simulink model "mpc1_sim_extended"  (R2020a)
settings: Solver=VariableStepAuto  StartTime=0.0  StopTime=10  RelTol=1e-3
values from neighbouring files (symbols this model uses):
  Ts = 0.1    [data_mpc.mat]    (also in so_priklad.m)
libraries: mpclib x3, cstblocks x3
settings Model: Creator=mgoubej  LastModifiedBy=mgoubej

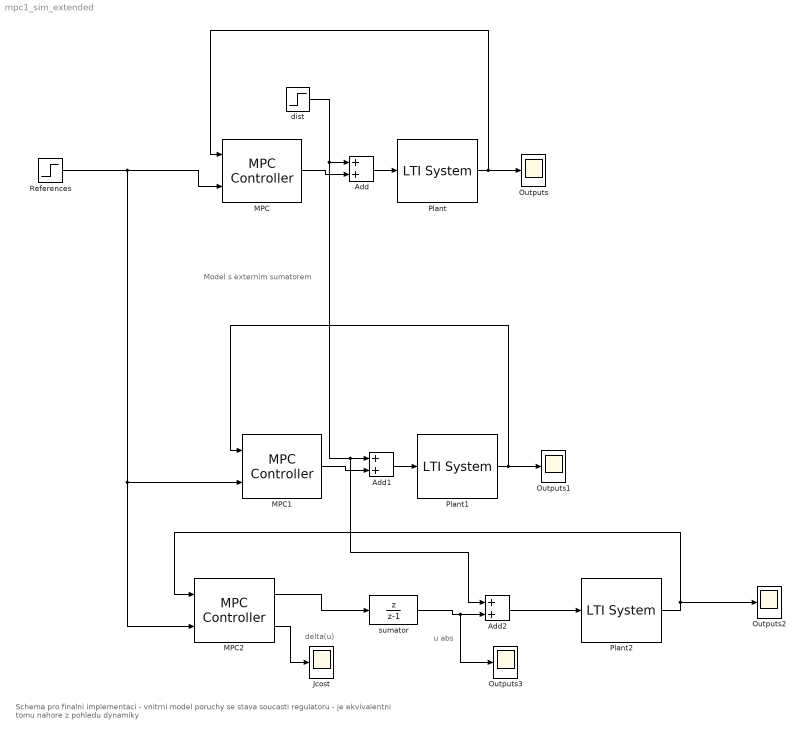
== system mpc1_sim_extended ==
  note: Schema pro finalni implementaci - vnitrni model poruchy se stava soucasti regulatoru - je ekvivalentni tomu nahore z pohledu dynamiky
  note: u abs
  note: delta(u)
  note: Model s externim sumatorem
  Add : Sum
  Add1 : Sum
  Add2 : Sum
  Jcost : Scope
  MPC : mpclib/MPC Controller  SCDEnableBlockLinearizationSpecification=on  mpcobj=mpc1_e  is_multiple=0  enable_value=0  return_u0=off  updateMPCinCallerWorkspace=on  md_inport=off  mv_inport=off  uref_inport=off  return_cost=off  return_mvseq=off  return_qpstatus=off  return_xseq=off  return_state=off  return_ovseq=off  state_inport=off  umin_inport=off  umax_inport=off  ymin_inport=off  ymax_inport=off  cc_inport=off  ywt_inport=off  uwt_inport=off  duwt_inport=off  rhoeps_inport=off  pm_inport=off  MaximumP=10  HorizonChoice=FixedHorizon  n_ts=0.1  n_p=10  n_mv=1  n_md=0  n_ud=0  n_mo=1  n_uo=0  BlockDataType=double  SampleTimeInherited=off  switch_inport=off
  MPC1 : mpclib/MPC Controller  SCDEnableBlockLinearizationSpecification=on  mpcobj=mpc1_e  is_multiple=0  enable_value=0  return_u0=off  updateMPCinCallerWorkspace=on  md_inport=off  mv_inport=off  uref_inport=off  return_cost=off  return_mvseq=off  return_qpstatus=off  return_xseq=off  return_state=off  return_ovseq=off  state_inport=off  umin_inport=off  umax_inport=off  ymin_inport=off  ymax_inport=off  cc_inport=off  ywt_inport=off  uwt_inport=off  duwt_inport=off  rhoeps_inport=off  pm_inport=off  MaximumP=10  HorizonChoice=FixedHorizon  n_ts=0.1  n_p=10  n_mv=1  n_md=0  n_ud=0  n_mo=1  n_uo=0  BlockDataType=double  SampleTimeInherited=off  switch_inport=off
  MPC2 : mpclib/MPC Controller  SCDEnableBlockLinearizationSpecification=on  mpcobj=mpc1_e  is_multiple=0  enable_value=0  return_u0=off  updateMPCinCallerWorkspace=on  md_inport=off  mv_inport=off  uref_inport=off  return_cost=on  return_mvseq=off  return_qpstatus=off  return_xseq=off  return_state=off  return_ovseq=off  state_inport=off  umin_inport=off  umax_inport=off  ymin_inport=off  ymax_inport=off  cc_inport=off  ywt_inport=off  uwt_inport=off  duwt_inport=off  rhoeps_inport=off  pm_inport=off  MaximumP=10  HorizonChoice=FixedHorizon  n_ts=0.1  n_p=10  n_mv=1  n_md=0  n_ud=0  n_mo=1  n_uo=0  BlockDataType=double  SampleTimeInherited=off  switch_inport=off
  Outputs{,1..3} (4 alike) : Scope
  Plant : cstblocks/LTI System  sys=Psse  IC=[]
  Plant1 : cstblocks/LTI System  sys=Psse  IC=[]
  Plant2 : cstblocks/LTI System  sys=Pss  IC=[]
  References : Step
  dist : Step  Time=5  After=0.1
  sumator : DiscreteTransferFcn  Numerator=[1 0]  Denominator=[1 -1]  SampleTime=Ts
  wires:
  References/1 -> MPC2/2, MPC1/2, MPC/2
  Plant/1 -> MPC/1, Outputs/1
  Add/1 -> Plant/1
  MPC/1 -> Add/2
  dist/1 -> Add2/1, Add1/1, Add/1
  MPC1/1 -> Add1/2
  Add1/1 -> Plant1/1
  Plant1/1 -> Outputs1/1, MPC1/1
  MPC2/1 -> sumator/1
  sumator/1 -> Outputs3/1, Add2/2
  Add2/1 -> Plant2/1
  Plant2/1 -> MPC2/1, Outputs2/1
  MPC2/2 -> Jcost/1
